simulink model "FaultCheck"  (R2022b)
settings: Solver=FixedStepAuto  StartTime=0.0  StopTime=10  FixedStep=1  RelTol=1e-3
undefined symbols (not defined in the file): C_Flt_IGBTULowerTempConfirmTh_u16, C_Flt_IGBTULowerTempDiagEn_b, C_Flt_IGBTULowerTempErrCode_u16, C_Flt_IGBTULowerTempPowerCoeff, C_Flt_IGBTULowerTempRecoveryTh_u16, C_Flt_IGBTULowerTempRecTh_s32, C_Flt_IGBTULowerTempTrigTh_s32, C_Flt_IGBTUOverTempConfirmTh_u16, C_Flt_IGBTUOverTempDiagEn_b, C_Flt_IGBTUOverTempErrCode_u16, C_Flt_IGBTUOverTempRecoveryTh_u16, C_Flt_IGBTUOverTempRecTh_s32, C_Flt_IGBTUOverTempTrigTh_s32, C_Flt_IGBTVLowerTempConfirmTh_u16, C_Flt_IGBTVLowerTempDiagEn_b, C_Flt_IGBTVLowerTempErrCode_u16, C_Flt_IGBTVLowerTempPowerCoeff, C_Flt_IGBTVLowerTempRecoveryTh_u16, C_Flt_IGBTVLowerTempRecTh_s32, C_Flt_IGBTVLowerTempTrigTh_s32, C_Flt_IGBTVOverTempConfirmTh_u16, C_Flt_IGBTVOverTempDiagEn_b, C_Flt_IGBTVOverTempErrCode_u16, C_Flt_IGBTVOverTempRecoveryTh_u16, C_Flt_IGBTVOverTempRecTh_s32, C_Flt_IGBTVOverTempTrigTh_s32, C_Flt_IGBTWLowerTempConfirmTh_u16, C_Flt_IGBTWLowerTempDiagEn_b, C_Flt_IGBTWLowerTempErrCode_u16, C_Flt_IGBTWLowerTempPowerCoeff, C_Flt_IGBTWLowerTempRecoveryTh_u16, C_Flt_IGBTWLowerTempRecTh_s32, C_Flt_IGBTWLowerTempTrigTh_s32, C_Flt_IGBTWOverTempConfirmTh_u16, C_Flt_IGBTWOverTempDiagEn_b, C_Flt_IGBTWOverTempErrCode_u16, C_Flt_IGBTWOverTempRecoveryTh_u16, C_Flt_IGBTWOverTempRecTh_s32, C_Flt_IGBTWOverTempTrigTh_s32, C_Flt_IuOCConfirmTh_u16, C_Flt_IuOCDiagEn_b, C_Flt_IuOCErrCode_u16, C_Flt_IuOCNegLimit_s32, C_Flt_IuOCPosLimit_s32, C_Flt_IuOCRecoveryTh_u16, C_Flt_IuZeroDriftDiagEn_b, C_Flt_IuZeroDriftErrCode_u16, C_Flt_IvOCConfirmTh_u16, C_Flt_IvOCDiagEn_b, C_Flt_IvOCErrCode_u16, C_Flt_IvOCNegLimit_s32, C_Flt_IvOCPosLimit_s32, C_Flt_IvOCRecoveryTh_u16, C_Flt_IvZeroDriftDiagEn_b, C_Flt_IvZeroDriftErrCode_u16, C_Flt_IwOCConfirmTh_u16, C_Flt_IwOCDiagEn_b, C_Flt_IwOCErrCode_u16, C_Flt_IwOCNegLimit_s32, C_Flt_IwOCPosLimit_s32 ... (+196)
libraries: YS_UserDefined_Library x21, simulink x5
(part 5 of 11)

== system FaultCheck/FaultDiagnose/IGBTTempDiag/IGBTWOverTempDiag/PowerReductionCoeffDeter ==
  IGBTWOverTempFltLevelOut : Inport
  PowerCoeff : Inport  Port=2
  If : If  IfExpression=u1 < 2  ElseIfExpressions=u1 == 2
  If Action Subsystem : Subsystem  TreatAsAtomicUnit=on
  If Action Subsystem1 : Subsystem  TreatAsAtomicUnit=on
  If Action Subsystem2 : Subsystem  TreatAsAtomicUnit=on
  Merge : Merge  Inputs=3
  IGBTWOverTempPowerCoeffOut : Outport
  wires:
  IGBTWOverTempFltLevelOut/1 -> If/1
  If/1 -> If Action Subsystem/Action
  If/2 -> If Action Subsystem1/Action
  If/3 -> If Action Subsystem2/Action
  PowerCoeff/1 -> If Action Subsystem1/1(PowerCoeff)
  If Action Subsystem/1(Coeff) -> Merge/1
  If Action Subsystem1/1(Coeff) -> Merge/2
  If Action Subsystem2/1(Coeff) -> Merge/3
  Merge/1 -> IGBTWOverTempPowerCoeffOut/1  "M_Flt_IGBTWOverTempPowerCoeffOut_s32"

== system FaultCheck/FaultDiagnose/MotorSpdFltDiag/MotorOverSpdOneNegDiag/Diagnose ==
  DiagEnOut : Inport
  MotorSpd : Inport  Port=2
  Parameter : Inport  Port=3
  Disable : Subsystem  TreatAsAtomicUnit=on
  If : If  IfExpression=u1 == 0
  Merge : Merge
  NormalDiag : Subsystem  TreatAsAtomicUnit=on
  MotorOverSpdOneNegFlgOut : Outport
  wires:
  DiagEnOut/1 -> If/1
  If/1 -> Disable/Action
  If/2 -> NormalDiag/Action
  MotorSpd/1 -> NormalDiag/1(MotorSpd)
  Parameter/1 -> NormalDiag/2(Parameter)
  Disable/1(MotorOverSpdOneNegFltDeb) -> Merge/1
  NormalDiag/1(MotorOverSpdOneNegFltDeb) -> Merge/2
  Merge/1 -> MotorOverSpdOneNegFlgOut/1  "M_Flt_MotorOverSpdOneNegFlgOut_b"

== system FaultCheck/FaultDiagnose/MotorSpdFltDiag/MotorOverSpdOneNegDiag/EnableJudgement ==
  SysSelfCheckDownFlg : Inport
  DiagEn : Inport  Port=2
  Constant : Constant  Value=true
  Logical Operator : Logic  AllPortsSameDT=off  OutDataTypeStr=boolean
  Logical Operator1 : Logic  AllPortsSameDT=off  OutDataTypeStr=boolean
  Logical Operator2 : Logic  AllPortsSameDT=off  OutDataTypeStr=boolean
  DiagEnOut : Outport
  wires:
  Logical Operator2/1 -> DiagEnOut/1  "M_Flt_MotorOverSpdOneNegDiagEn_b"
  Logical Operator/1 -> Logical Operator2/1
  SysSelfCheckDownFlg/1 -> Logical Operator/2
  DiagEn/1 -> Logical Operator1/2
  Constant/1 -> Logical Operator/1, Logical Operator1/1
  Logical Operator1/1 -> Logical Operator2/2

== system FaultCheck/FaultDiagnose/MotorSpdFltDiag/MotorOverSpdOneNegDiag/FaultLevelDeter ==
  MotorOverSpdOneNegFlgOut : Inport
  FaultLevel : Inport  Port=2
  If : If  IfExpression=u1 == 0
  LowerOne : Subsystem  TreatAsAtomicUnit=on
  Merge : Merge
  Normal : Subsystem  TreatAsAtomicUnit=on
  MotorOverSpdOneNegFltLevelOut : Outport
  wires:
  MotorOverSpdOneNegFlgOut/1 -> If/1
  If/1 -> Normal/Action
  If/2 -> LowerOne/Action
  Normal/1(MotorOverSpdOneNegFltLevel) -> Merge/1
  LowerOne/1(MotorOverSpdOneNegFltLevel) -> Merge/2
  Merge/1 -> MotorOverSpdOneNegFltLevelOut/1  "M_Flt_MotorOverSpdOneNegFltLevelOut_u8"
  FaultLevel/1 -> LowerOne/1(FaultLevel)

== system FaultCheck/FaultDiagnose/MotorSpdFltDiag/MotorOverSpdOneNegDiag/Parameters ==
  MotorSpd : Inport
  1-D Lookup Table1 : Lookup_n-D  NumberOfTableDimensions=1  BreakpointsForDimension1=[-5:5]  BreakpointsForDimension1DataTypeStr=Inherit: Inherit from 'Breakpoint data'  IndexSearchMethod=Linear search  Table=tanh([-5:5])  TableDataTypeStr=Inherit: Inherit from 'Table data'  ExtrapMethod=Clip  UseLastTableValue=on  InternalRulePriority=Speed  OutDataTypeStr=single  RndMeth=Simplest
  Bus Creator : BusCreator  Inputs=8
  Constant : Constant  Value=C_Flt_MotorOverSpdOneNegTrigTh_s32
  Constant1 : Constant  Value=C_Flt_MotorOverSpdOneNegRecTh_s32
  Constant10 : Constant  Value=C_Flt_MotorOverSpdOneNegRecoveryTh_u16
  Constant11 : Constant  Value=C_Flt_LevelTwo_u8
  Constant7 : Constant  Value=C_Flt_MotorOverSpdOneNegDiagEn_b
  Constant8 : Constant  Value=C_Flt_MotorOverSpdOneNegErrCode_u16
  Constant9 : Constant  Value=C_Flt_MotorOverSpdOneNegConfirmTh_u16
  Param : Outport
  wires:
  Bus Creator/1 -> Param/1
  MotorSpd/1 -> 1-D Lookup Table1/1
  Constant/1 -> Bus Creator/1  "MotorOverSpdOneNegTrigTh"
  Constant7/1 -> Bus Creator/3  "MotorOverSpdOneNegDiagEn"
  Constant8/1 -> Bus Creator/4  "MotorOverSpdOneNegErrCode"
  Constant9/1 -> Bus Creator/5  "MotorOverSpdOneNegConfirmTh"
  Constant10/1 -> Bus Creator/6  "MotorOverSpdOneNegRecoveryTh"
  Constant11/1 -> Bus Creator/7  "MotorOverSpdOneNegFltLevel"
  1-D Lookup Table1/1 -> Bus Creator/8  "MotorOverSpdOneNegPowerCoeff"
  Constant1/1 -> Bus Creator/2  "MotorOverSpdOneNegRecTh"

== system FaultCheck/FaultDiagnose/MotorSpdFltDiag/MotorOverSpdOneNegDiag/PowerReductionCoeffDeter ==
  MotorOverSpdOneNegFltLevelOut : Inport
  PowerCoeff : Inport  Port=2
  If : If  IfExpression=u1 < 2  ElseIfExpressions=u1 == 2
  If Action Subsystem : Subsystem  TreatAsAtomicUnit=on
  If Action Subsystem1 : Subsystem  TreatAsAtomicUnit=on
  If Action Subsystem2 : Subsystem  TreatAsAtomicUnit=on
  Merge : Merge  Inputs=3
  MotorOverSpdOneNegPowerCoeffOut : Outport
  wires:
  MotorOverSpdOneNegFltLevelOut/1 -> If/1
  If/1 -> If Action Subsystem/Action
  If/2 -> If Action Subsystem1/Action
  If/3 -> If Action Subsystem2/Action
  PowerCoeff/1 -> If Action Subsystem1/1(PowerCoeff)
  If Action Subsystem/1(Coeff) -> Merge/1
  If Action Subsystem1/1(Coeff) -> Merge/2
  If Action Subsystem2/1(Coeff) -> Merge/3
  Merge/1 -> MotorOverSpdOneNegPowerCoeffOut/1  "M_Flt_MotorOverSpdOneNegPowerCoeffOut_s32"

== system FaultCheck/FaultDiagnose/MotorSpdFltDiag/MotorOverSpdOnePosDiag/Diagnose ==
  DiagEnOut : Inport
  MotorSpd : Inport  Port=2
  Parameter : Inport  Port=3
  Disable : Subsystem  TreatAsAtomicUnit=on
  If : If  IfExpression=u1 == 0
  Merge : Merge
  NormalDiag : Subsystem  TreatAsAtomicUnit=on
  MotorOverSpdOnePosFlgOut : Outport
  wires:
  DiagEnOut/1 -> If/1
  If/1 -> Disable/Action
  If/2 -> NormalDiag/Action
  MotorSpd/1 -> NormalDiag/1(MotorSpd)
  Parameter/1 -> NormalDiag/2(Parameter)
  Disable/1(MotorOverSpdOnePosFltDeb) -> Merge/1
  NormalDiag/1(MotorOverSpdOnePosFltDeb) -> Merge/2
  Merge/1 -> MotorOverSpdOnePosFlgOut/1  "M_Flt_MotorOverSpdOnePosFlgOut_b"

== system FaultCheck/FaultDiagnose/MotorSpdFltDiag/MotorOverSpdOnePosDiag/EnableJudgement ==
  SysSelfCheckDownFlg : Inport
  DiagEn : Inport  Port=2
  Constant : Constant  Value=true
  Logical Operator : Logic  AllPortsSameDT=off  OutDataTypeStr=boolean
  Logical Operator1 : Logic  AllPortsSameDT=off  OutDataTypeStr=boolean
  Logical Operator2 : Logic  AllPortsSameDT=off  OutDataTypeStr=boolean
  DiagEnOut : Outport
  wires:
  Logical Operator2/1 -> DiagEnOut/1  "M_Flt_MotorOverSpdOnePosDiagEn_b"
  Logical Operator/1 -> Logical Operator2/1
  SysSelfCheckDownFlg/1 -> Logical Operator/2
  DiagEn/1 -> Logical Operator1/2
  Constant/1 -> Logical Operator/1, Logical Operator1/1
  Logical Operator1/1 -> Logical Operator2/2

== system FaultCheck/FaultDiagnose/MotorSpdFltDiag/MotorOverSpdOnePosDiag/FaultLevelDeter ==
  MotorOverSpdOnePosFlgOut : Inport
  FaultLevel : Inport  Port=2
  If : If  IfExpression=u1 == 0
  LowerOne : Subsystem  TreatAsAtomicUnit=on
  Merge : Merge
  Normal : Subsystem  TreatAsAtomicUnit=on
  MotorOverSpdOnePosFltLevelOut : Outport
  wires:
  MotorOverSpdOnePosFlgOut/1 -> If/1
  If/1 -> Normal/Action
  If/2 -> LowerOne/Action
  Normal/1(MotorOverSpdOnePosFltLevel) -> Merge/1
  LowerOne/1(MotorOverSpdOnePosFltLevel) -> Merge/2
  Merge/1 -> MotorOverSpdOnePosFltLevelOut/1  "M_Flt_MotorOverSpdOnePosFltLevelOut_u8"
  FaultLevel/1 -> LowerOne/1(FaultLevel)

== system FaultCheck/FaultDiagnose/MotorSpdFltDiag/MotorOverSpdOnePosDiag/Parameters ==
  MotorSpd : Inport
  1-D Lookup Table1 : Lookup_n-D  NumberOfTableDimensions=1  BreakpointsForDimension1=[-5:5]  BreakpointsForDimension1DataTypeStr=Inherit: Inherit from 'Breakpoint data'  IndexSearchMethod=Linear search  Table=tanh([-5:5])  TableDataTypeStr=Inherit: Inherit from 'Table data'  ExtrapMethod=Clip  UseLastTableValue=on  InternalRulePriority=Speed  OutDataTypeStr=single  RndMeth=Simplest
  Bus Creator : BusCreator  Inputs=8
  Constant : Constant  Value=C_Flt_MotorOverSpdOnePosTrigTh_s32
  Constant1 : Constant  Value=C_Flt_MotorOverSpdOnePosRecTh_s32
  Constant10 : Constant  Value=C_Flt_MotorOverSpdOnePosRecoveryTh_u16
  Constant11 : Constant  Value=C_Flt_LevelTwo_u8
  Constant7 : Constant  Value=C_Flt_MotorOverSpdOnePosDiagEn_b
  Constant8 : Constant  Value=C_Flt_MotorOverSpdOnePosErrCode_u16
  Constant9 : Constant  Value=C_Flt_MotorOverSpdOnePosConfirmTh_u16
  Param : Outport
  wires:
  Bus Creator/1 -> Param/1
  MotorSpd/1 -> 1-D Lookup Table1/1
  Constant/1 -> Bus Creator/1  "MotorOverSpdOnePosTrigTh"
  Constant7/1 -> Bus Creator/3  "MotorOverSpdOnePosDiagEn"
  Constant8/1 -> Bus Creator/4  "MotorOverSpdOnePosErrCode"
  Constant9/1 -> Bus Creator/5  "MotorOverSpdOnePosConfirmTh"
  Constant10/1 -> Bus Creator/6  "MotorOverSpdOnePosRecoveryTh"
  Constant11/1 -> Bus Creator/7  "MotorOverSpdOnePosFltLevel"
  1-D Lookup Table1/1 -> Bus Creator/8  "MotorOverSpdOnePosPowerCoeff"
  Constant1/1 -> Bus Creator/2  "MotorOverSpdOnePosRecTh"

== system FaultCheck/FaultDiagnose/MotorSpdFltDiag/MotorOverSpdOnePosDiag/PowerReductionCoeffDeter ==
  MotorOverSpdOnePosFltLevelOut : Inport
  PowerCoeff : Inport  Port=2
  If : If  IfExpression=u1 < 2  ElseIfExpressions=u1 == 2
  If Action Subsystem : Subsystem  TreatAsAtomicUnit=on
  If Action Subsystem1 : Subsystem  TreatAsAtomicUnit=on
  If Action Subsystem2 : Subsystem  TreatAsAtomicUnit=on
  Merge : Merge  Inputs=3
  MotorOverSpdOnePosPowerCoeffOut : Outport
  wires:
  MotorOverSpdOnePosFltLevelOut/1 -> If/1
  If/1 -> If Action Subsystem/Action
  If/2 -> If Action Subsystem1/Action
  If/3 -> If Action Subsystem2/Action
  PowerCoeff/1 -> If Action Subsystem1/1(PowerCoeff)
  If Action Subsystem/1(Coeff) -> Merge/1
  If Action Subsystem1/1(Coeff) -> Merge/2
  If Action Subsystem2/1(Coeff) -> Merge/3
  Merge/1 -> MotorOverSpdOnePosPowerCoeffOut/1  "M_Flt_MotorOverSpdOnePosPowerCoeffOut_s32"

== system FaultCheck/FaultDiagnose/MotorSpdFltDiag/MotorOverSpdTwoNegDiag/Diagnose ==
  DiagEnOut : Inport
  MotorSpd : Inport  Port=2
  Parameter : Inport  Port=3
  Disable : Subsystem  TreatAsAtomicUnit=on
  If : If  IfExpression=u1 == 0
  Merge : Merge
  NormalDiag : Subsystem  TreatAsAtomicUnit=on
  MotorOverSpdTwoNegFlgOut : Outport
  wires:
  Merge/1 -> MotorOverSpdTwoNegFlgOut/1  "M_Flt_MotorOverSpdTwoNegFlgOut_b"
  NormalDiag/1(MotorOverSpdTwoNegFltDeb) -> Merge/2
  Disable/1(MotorOverSpdTwoNegFltDeb) -> Merge/1
  Parameter/1 -> NormalDiag/2(Parameter)
  MotorSpd/1 -> NormalDiag/1(PCBTemp)
  If/2 -> NormalDiag/Action
  If/1 -> Disable/Action
  DiagEnOut/1 -> If/1

== system FaultCheck/FaultDiagnose/MotorSpdFltDiag/MotorOverSpdTwoNegDiag/EnableJudgement ==
  SysSelfCheckDownFlg : Inport
  DiagEn : Inport  Port=2
  Constant : Constant  Value=true
  Logical Operator : Logic  AllPortsSameDT=off  OutDataTypeStr=boolean
  Logical Operator1 : Logic  AllPortsSameDT=off  OutDataTypeStr=boolean
  Logical Operator2 : Logic  AllPortsSameDT=off  OutDataTypeStr=boolean
  DiagEnOut : Outport
  wires:
  Logical Operator1/1 -> Logical Operator2/2
  Constant/1 -> Logical Operator1/1, Logical Operator/1
  DiagEn/1 -> Logical Operator1/2
  SysSelfCheckDownFlg/1 -> Logical Operator/2
  Logical Operator/1 -> Logical Operator2/1
  Logical Operator2/1 -> DiagEnOut/1  "M_Flt_MotorOverSpdTwoNegDiagEn_b"

== system FaultCheck/FaultDiagnose/MotorSpdFltDiag/MotorOverSpdTwoNegDiag/FaultLevelDeter ==
  MotorOverSpdTwoNegFlgOut : Inport
  FaultLevel : Inport  Port=2
  If : If  IfExpression=u1 == 0
  LowerOne : Subsystem  TreatAsAtomicUnit=on
  Merge : Merge
  Normal : Subsystem  TreatAsAtomicUnit=on
  MotorOverSpdTwoNegFltLevelOut : Outport
  wires:
  FaultLevel/1 -> LowerOne/1(FaultLevel)
  Merge/1 -> MotorOverSpdTwoNegFltLevelOut/1  "M_Flt_MotorOverSpdTwoNegFltLevelOut_u8"
  LowerOne/1(MotorOverSpdTwoNegFltLevel) -> Merge/2
  Normal/1(MotorOverSpdTwoNegFltLevel) -> Merge/1
  If/2 -> LowerOne/Action
  If/1 -> Normal/Action
  MotorOverSpdTwoNegFlgOut/1 -> If/1

== system FaultCheck/FaultDiagnose/MotorSpdFltDiag/MotorOverSpdTwoNegDiag/Parameters ==
  Bus Creator : BusCreator  Inputs=8
  Constant : Constant  Value=C_Flt_MotorOverSpdTwoNegTrigTh_s32
  Constant1 : Constant  Value=C_Flt_MotorOverSpdTwoNegRecTh_s32
  Constant10 : Constant  Value=C_Flt_MotorOverSpdTwoNegRecoveryTh_u16
  Constant11 : Constant  Value=C_Flt_LevelThree_u8
  Constant2 : Constant  Value=C_Flt_PowerCoeffZero_s32
  Constant7 : Constant  Value=C_Flt_MotorOverSpdTwoNegDiagEn_b
  Constant8 : Constant  Value=C_Flt_MotorOverSpdTwoNegErrCode_u16
  Constant9 : Constant  Value=C_Flt_MotorOverSpdTwoNegConfirmTh_u16
  Param : Outport
  wires:
  Constant1/1 -> Bus Creator/2  "MotorOverSpdTwoNegRecTh"
  Constant2/1 -> Bus Creator/8  "MotorOverSpdTwoNegPowerCoeff"
  Constant11/1 -> Bus Creator/7  "MotorOverSpdTwoNegFltLevel"
  Constant10/1 -> Bus Creator/6  "MotorOverSpdTwoNegRecoveryTh"
  Constant9/1 -> Bus Creator/5  "MotorOverSpdTwoNegConfirmTh"
  Constant8/1 -> Bus Creator/4  "MotorOverSpdTwoNegErrCode"
  Constant7/1 -> Bus Creator/3  "MotorOverSpdTwoNegDiagEn"
  Constant/1 -> Bus Creator/1  "MotorOverSpdTwoNegTrigTh"
  Bus Creator/1 -> Param/1

== system FaultCheck/FaultDiagnose/MotorSpdFltDiag/MotorOverSpdTwoNegDiag/PowerReductionCoeffDeter ==
  MotorOverSpdTwoNegFltLevelOut : Inport
  PowerCoeff : Inport  Port=2
  If : If  IfExpression=u1 < 2  ElseIfExpressions=u1 == 2
  If Action Subsystem : Subsystem  TreatAsAtomicUnit=on
  If Action Subsystem1 : Subsystem  TreatAsAtomicUnit=on
  If Action Subsystem2 : Subsystem  TreatAsAtomicUnit=on
  Merge : Merge  Inputs=3
  MotorOverSpdTwoNegPowerCoeffOut : Outport
  wires:
  Merge/1 -> MotorOverSpdTwoNegPowerCoeffOut/1  "M_Flt_MotorOverSpdTwoNegPowerCoeffOut_s32"
  If Action Subsystem2/1(Coeff) -> Merge/3
  If Action Subsystem1/1(Coeff) -> Merge/2
  If Action Subsystem/1(Coeff) -> Merge/1
  PowerCoeff/1 -> If Action Subsystem1/1(PowerCoeff)
  If/3 -> If Action Subsystem2/Action
  If/2 -> If Action Subsystem1/Action
  If/1 -> If Action Subsystem/Action
  MotorOverSpdTwoNegFltLevelOut/1 -> If/1

== system FaultCheck/FaultDiagnose/MotorSpdFltDiag/MotorOverSpdTwoPosDiag/Diagnose ==
  DiagEnOut : Inport
  MotorSpd : Inport  Port=2
  Parameter : Inport  Port=3
  Disable : Subsystem  TreatAsAtomicUnit=on
  If : If  IfExpression=u1 == 0
  Merge : Merge
  NormalDiag : Subsystem  TreatAsAtomicUnit=on
  MotorOverSpdTwoPosFlgOut : Outport
  wires:
  Merge/1 -> MotorOverSpdTwoPosFlgOut/1  "M_Flt_MotorOverSpdTwoPosFlgOut_b"
  NormalDiag/1(MotorOverSpdTwoPosFltDeb) -> Merge/2
  Disable/1(MotorOverSpdTwoPosFltDeb) -> Merge/1
  Parameter/1 -> NormalDiag/2(Parameter)
  MotorSpd/1 -> NormalDiag/1(MotorSpd)
  If/2 -> NormalDiag/Action
  If/1 -> Disable/Action
  DiagEnOut/1 -> If/1

== system FaultCheck/FaultDiagnose/MotorSpdFltDiag/MotorOverSpdTwoPosDiag/EnableJudgement ==
  SysSelfCheckDownFlg : Inport
  DiagEn : Inport  Port=2
  Constant : Constant  Value=true
  Logical Operator : Logic  AllPortsSameDT=off  OutDataTypeStr=boolean
  Logical Operator1 : Logic  AllPortsSameDT=off  OutDataTypeStr=boolean
  Logical Operator2 : Logic  AllPortsSameDT=off  OutDataTypeStr=boolean
  DiagEnOut : Outport
  wires:
  Logical Operator1/1 -> Logical Operator2/2
  Constant/1 -> Logical Operator1/1, Logical Operator/1
  DiagEn/1 -> Logical Operator1/2
  SysSelfCheckDownFlg/1 -> Logical Operator/2
  Logical Operator/1 -> Logical Operator2/1
  Logical Operator2/1 -> DiagEnOut/1  "M_Flt_MotorOverSpdTwoPosDiagEn_b"

== system FaultCheck/FaultDiagnose/MotorSpdFltDiag/MotorOverSpdTwoPosDiag/FaultLevelDeter ==
  MotorOverSpdTwoPosFlgOut : Inport
  FaultLevel : Inport  Port=2
  If : If  IfExpression=u1 == 0
  LowerOne : Subsystem  TreatAsAtomicUnit=on
  Merge : Merge
  Normal : Subsystem  TreatAsAtomicUnit=on
  MotorOverSpdTwoPosFltLevelOut : Outport
  wires:
  FaultLevel/1 -> LowerOne/1(FaultLevel)
  Merge/1 -> MotorOverSpdTwoPosFltLevelOut/1  "M_Flt_MotorOverSpdTwoPosFltLevelOut_u8"
  LowerOne/1(MotorOverSpdTwoPosFltLevel) -> Merge/2
  Normal/1(MotorOverSpdTwoPosFltLevel) -> Merge/1
  If/2 -> LowerOne/Action
  If/1 -> Normal/Action
  MotorOverSpdTwoPosFlgOut/1 -> If/1

== system FaultCheck/FaultDiagnose/MotorSpdFltDiag/MotorOverSpdTwoPosDiag/Parameters ==
  Bus Creator : BusCreator  Inputs=8
  Constant : Constant  Value=C_Flt_MotorOverSpdTwoPosTrigTh_s32
  Constant1 : Constant  Value=C_Flt_MotorOverSpdTwoPosRecTh_s32
  Constant10 : Constant  Value=C_Flt_MotorOverSpdTwoPosRecoveryTh_u16
  Constant11 : Constant  Value=C_Flt_LevelThree_u8
  Constant2 : Constant  Value=C_Flt_PowerCoeffZero_s32
  Constant7 : Constant  Value=C_Flt_MotorOverSpdTwoPosDiagEn_b
  Constant8 : Constant  Value=C_Flt_MotorOverSpdTwoPosErrCode_u16
  Constant9 : Constant  Value=C_Flt_MotorOverSpdTwoPosConfirmTh_u16
  Param : Outport
  wires:
  Constant1/1 -> Bus Creator/2  "MotorOverSpdTwoPosRecTh"
  Constant2/1 -> Bus Creator/8  "MotorOverSpdTwoPosPowerCoeff"
  Constant11/1 -> Bus Creator/7  "MotorOverSpdTwoPosFltLevel"
  Constant10/1 -> Bus Creator/6  "MotorOverSpdTwoPosRecoveryTh"
  Constant9/1 -> Bus Creator/5  "MotorOverSpdTwoPosConfirmTh"
  Constant8/1 -> Bus Creator/4  "MotorOverSpdTwoPosErrCode"
  Constant7/1 -> Bus Creator/3  "MotorOverSpdTwoPosDiagEn"
  Constant/1 -> Bus Creator/1  "MotorOverSpdTwoPosTrigTh"
  Bus Creator/1 -> Param/1

== system FaultCheck/FaultDiagnose/MotorSpdFltDiag/MotorOverSpdTwoPosDiag/PowerReductionCoeffDeter ==
  MotorOverSpdTwoPosFltLevelOut : Inport
  PowerCoeff : Inport  Port=2
  If : If  IfExpression=u1 < 2  ElseIfExpressions=u1 == 2
  If Action Subsystem : Subsystem  TreatAsAtomicUnit=on
  If Action Subsystem1 : Subsystem  TreatAsAtomicUnit=on
  If Action Subsystem2 : Subsystem  TreatAsAtomicUnit=on
  Merge : Merge  Inputs=3
  MotorOverSpdTwoPosPowerCoeffOut : Outport
  wires:
  Merge/1 -> MotorOverSpdTwoPosPowerCoeffOut/1  "M_Flt_MotorOverSpdTwoPosPowerCoeffOut_s32"
  If Action Subsystem2/1(Coeff) -> Merge/3
  If Action Subsystem1/1(Coeff) -> Merge/2
  If Action Subsystem/1(Coeff) -> Merge/1
  PowerCoeff/1 -> If Action Subsystem1/1(PowerCoeff)
  If/3 -> If Action Subsystem2/Action
  If/2 -> If Action Subsystem1/Action
  If/1 -> If Action Subsystem/Action
  MotorOverSpdTwoPosFltLevelOut/1 -> If/1

== system FaultCheck/FaultDiagnose/MotorTempDiag/MotorLowerTempDiag/Diagnose ==
  DiagEnOut : Inport
  MotorTemp : Inport  Port=2
  Parameter : Inport  Port=3
  Disable : Subsystem  TreatAsAtomicUnit=on
  If : If  IfExpression=u1 == 0
  Merge : Merge
  NormalDiag : Subsystem  TreatAsAtomicUnit=on
  MotorLowerTempFlgOut : Outport
  wires:
  Merge/1 -> MotorLowerTempFlgOut/1  "M_Flt_MotorLowerTempFlgOut_b"
  NormalDiag/1(MotorLowerTempFltDeb) -> Merge/2
  Disable/1(MotorLowerTempFltDeb) -> Merge/1
  Parameter/1 -> NormalDiag/2(Parameter)
  MotorTemp/1 -> NormalDiag/1(MotorTemp)
  If/2 -> NormalDiag/Action
  If/1 -> Disable/Action
  DiagEnOut/1 -> If/1

== system FaultCheck/FaultDiagnose/MotorTempDiag/MotorLowerTempDiag/EnableJudgement ==
  SysSelfCheckDownFlg : Inport
  DiagEn : Inport  Port=2
  Constant : Constant  Value=true
  Logical Operator : Logic  AllPortsSameDT=off  OutDataTypeStr=boolean
  Logical Operator1 : Logic  AllPortsSameDT=off  OutDataTypeStr=boolean
  Logical Operator2 : Logic  AllPortsSameDT=off  OutDataTypeStr=boolean
  DiagEnOut : Outport
  wires:
  Logical Operator1/1 -> Logical Operator2/2
  Constant/1 -> Logical Operator1/1, Logical Operator/1
  DiagEn/1 -> Logical Operator1/2
  SysSelfCheckDownFlg/1 -> Logical Operator/2
  Logical Operator/1 -> Logical Operator2/1
  Logical Operator2/1 -> DiagEnOut/1  "M_Flt_MotorLowerTempDiagEn_b"

== system FaultCheck/FaultDiagnose/MotorTempDiag/MotorLowerTempDiag/FaultLevelDeter ==
  MotorLowerTempFlgOut : Inport
  FaultLevel : Inport  Port=2
  If : If  IfExpression=u1 == 0
  LowerOne : Subsystem  TreatAsAtomicUnit=on
  Merge : Merge
  Normal : Subsystem  TreatAsAtomicUnit=on
  MotorLowerTempFltLevelOut : Outport
  wires:
  FaultLevel/1 -> LowerOne/1(FaultLevel)
  Merge/1 -> MotorLowerTempFltLevelOut/1  "M_Flt_MotorLowerTempFltLevelOut_u8"
  LowerOne/1(MotorLowerTempFltLevel) -> Merge/2
  Normal/1(MotorLowerTempFltLevel) -> Merge/1
  If/2 -> LowerOne/Action
  If/1 -> Normal/Action
  MotorLowerTempFlgOut/1 -> If/1

== system FaultCheck/FaultDiagnose/MotorTempDiag/MotorLowerTempDiag/Parameters ==
  Bus Creator : BusCreator  Inputs=8
  Constant : Constant  Value=C_Flt_MotorLowerTempTrigTh_s32
  Constant1 : Constant  Value=C_Flt_MotorLowerTempRecTh_s32
  Constant10 : Constant  Value=C_Flt_MotorLowerTempRecoveryTh_u16
  Constant11 : Constant  Value=C_Flt_LevelTwo_u8
  Constant2 : Constant  Value=C_Flt_MotorLowerTempPowerCoeff
  Constant7 : Constant  Value=C_Flt_MotorLowerTempDiagEn_b
  Constant8 : Constant  Value=C_Flt_MotorLowerTempErrCode_u16
  Constant9 : Constant  Value=C_Flt_MotorLowerTempConfirmTh_u16
  Param : Outport
  wires:
  Constant1/1 -> Bus Creator/2  "MotorLowerTempRecTh"
  Constant2/1 -> Bus Creator/8  "MotorLowerTempPowerCoeff"
  Constant11/1 -> Bus Creator/7  "MotorLowerTempFltLevel"
  Constant10/1 -> Bus Creator/6  "MotorLowerTempRecoveryTh"
  Constant9/1 -> Bus Creator/5  "MotorLowerTempConfirmTh"
  Constant8/1 -> Bus Creator/4  "MotorLowerTempErrCode"
  Constant7/1 -> Bus Creator/3  "MotorLowerTempDiagEn"
  Constant/1 -> Bus Creator/1  "MotorLowerTempTrigTh"
  Bus Creator/1 -> Param/1

== system FaultCheck/FaultDiagnose/MotorTempDiag/MotorLowerTempDiag/PowerReductionCoeffDeter ==
  MotorLowerTempFltLevelOut : Inport
  PowerCoeff : Inport  Port=2
  If : If  IfExpression=u1 < 2  ElseIfExpressions=u1 == 2
  If Action Subsystem : Subsystem  TreatAsAtomicUnit=on
  If Action Subsystem1 : Subsystem  TreatAsAtomicUnit=on
  If Action Subsystem2 : Subsystem  TreatAsAtomicUnit=on
  Merge : Merge  Inputs=3
  MotorLowerTempPowerCoeffOut : Outport
  wires:
  Merge/1 -> MotorLowerTempPowerCoeffOut/1  "M_Flt_MotorLowerTempPowerCoeffOut_s32"
  If Action Subsystem2/1(Coeff) -> Merge/3
  If Action Subsystem1/1(Coeff) -> Merge/2
  If Action Subsystem/1(Coeff) -> Merge/1
  PowerCoeff/1 -> If Action Subsystem1/1(PowerCoeff)
  If/3 -> If Action Subsystem2/Action
  If/2 -> If Action Subsystem1/Action
  If/1 -> If Action Subsystem/Action
  MotorLowerTempFltLevelOut/1 -> If/1

== system FaultCheck/FaultDiagnose/MotorTempDiag/MotorOverTempDiag/Diagnose ==
  DiagEnOut : Inport
  MotorTemp : Inport  Port=2
  Parameter : Inport  Port=3
  Disable : Subsystem  TreatAsAtomicUnit=on
  If : If  IfExpression=u1 == 0
  Merge : Merge
  NormalDiag : Subsystem  TreatAsAtomicUnit=on
  MotorOverTempFlgOut : Outport
  wires:
  DiagEnOut/1 -> If/1
  If/1 -> Disable/Action
  If/2 -> NormalDiag/Action
  MotorTemp/1 -> NormalDiag/1(MotorTemp)
  Parameter/1 -> NormalDiag/2(Parameter)
  Disable/1(MotorOverTempFltDeb) -> Merge/1
  NormalDiag/1(MotorOverTempFltDeb) -> Merge/2
  Merge/1 -> MotorOverTempFlgOut/1  "M_Flt_MotorOverTempFlgOut_b"

== system FaultCheck/FaultDiagnose/MotorTempDiag/MotorOverTempDiag/EnableJudgement ==
  SysSelfCheckDownFlg : Inport
  DiagEn : Inport  Port=2
  Constant : Constant  Value=true
  Logical Operator : Logic  AllPortsSameDT=off  OutDataTypeStr=boolean
  Logical Operator1 : Logic  AllPortsSameDT=off  OutDataTypeStr=boolean
  Logical Operator2 : Logic  AllPortsSameDT=off  OutDataTypeStr=boolean
  DiagEnOut : Outport
  wires:
  Logical Operator2/1 -> DiagEnOut/1  "M_Flt_MotorOverTempDiagEn_b"
  Logical Operator/1 -> Logical Operator2/1
  SysSelfCheckDownFlg/1 -> Logical Operator/2
  DiagEn/1 -> Logical Operator1/2
  Constant/1 -> Logical Operator/1, Logical Operator1/1
  Logical Operator1/1 -> Logical Operator2/2

== system FaultCheck/FaultDiagnose/MotorTempDiag/MotorOverTempDiag/FaultLevelDeter ==
  MotorOverTempFlgOut : Inport
  FaultLevel : Inport  Port=2
  If : If  IfExpression=u1 == 0
  LowerOne : Subsystem  TreatAsAtomicUnit=on
  Merge : Merge
  Normal : Subsystem  TreatAsAtomicUnit=on
  MotorOverTempFltLevelOut : Outport
  wires:
  MotorOverTempFlgOut/1 -> If/1
  If/1 -> Normal/Action
  If/2 -> LowerOne/Action
  Normal/1(MotorOverTempFltLevel) -> Merge/1
  LowerOne/1(MotorOverTempFltLevel) -> Merge/2
  Merge/1 -> MotorOverTempFltLevelOut/1  "M_Flt_MotorOverTempFltLevelOut_u8"
  FaultLevel/1 -> LowerOne/1(FaultLevel)

== system FaultCheck/FaultDiagnose/MotorTempDiag/MotorOverTempDiag/Parameters ==
  MotorTemp : Inport
  1-D Lookup Table1 : Lookup_n-D  NumberOfTableDimensions=1  BreakpointsForDimension1=[-5:5]  BreakpointsForDimension1DataTypeStr=Inherit: Inherit from 'Breakpoint data'  IndexSearchMethod=Linear search  Table=tanh([-5:5])  TableDataTypeStr=Inherit: Inherit from 'Table data'  ExtrapMethod=Clip  UseLastTableValue=on  InternalRulePriority=Speed  OutDataTypeStr=single  RndMeth=Simplest
  Bus Creator : BusCreator  Inputs=8
  Constant : Constant  Value=C_Flt_MotorOverTempTrigTh_s32
  Constant1 : Constant  Value=C_Flt_MotorOverTempRecTh_s32
  Constant10 : Constant  Value=C_Flt_MotorOverTempRecoveryTh_u16
  Constant11 : Constant  Value=C_Flt_LevelTwo_u8
  Constant7 : Constant  Value=C_Flt_MotorOverTempDiagEn_b
  Constant8 : Constant  Value=C_Flt_MotorOverTempErrCode_u16
  Constant9 : Constant  Value=C_Flt_MotorOverTempConfirmTh_u16
  Param : Outport
  wires:
  Bus Creator/1 -> Param/1
  MotorTemp/1 -> 1-D Lookup Table1/1
  Constant/1 -> Bus Creator/1  "MotorOverTempTrigTh"
  Constant7/1 -> Bus Creator/3  "MotorOverTempDiagEn"
  Constant8/1 -> Bus Creator/4  "MotorOverTempErrCode"
  Constant9/1 -> Bus Creator/5  "MotorOverTempConfirmTh"
  Constant10/1 -> Bus Creator/6  "MotorOverTempRecoveryTh"
  Constant11/1 -> Bus Creator/7  "MotorOverTempFltLevel"
  1-D Lookup Table1/1 -> Bus Creator/8  "MotorOverTempPowerCoeff"
  Constant1/1 -> Bus Creator/2  "MotorOverTempRecTh"

== system FaultCheck/FaultDiagnose/MotorTempDiag/MotorOverTempDiag/PowerReductionCoeffDeter ==
  MotorOverTempFltLevelOut : Inport
  PowerCoeff : Inport  Port=2
  If : If  IfExpression=u1 < 2  ElseIfExpressions=u1 == 2
  If Action Subsystem : Subsystem  TreatAsAtomicUnit=on
  If Action Subsystem1 : Subsystem  TreatAsAtomicUnit=on
  If Action Subsystem2 : Subsystem  TreatAsAtomicUnit=on
  Merge : Merge  Inputs=3
  MotorOverTempPowerCoeffOut : Outport
  wires:
  MotorOverTempFltLevelOut/1 -> If/1
  If/1 -> If Action Subsystem/Action
  If/2 -> If Action Subsystem1/Action
  If/3 -> If Action Subsystem2/Action
  PowerCoeff/1 -> If Action Subsystem1/1(PowerCoeff)
  If Action Subsystem/1(Coeff) -> Merge/1
  If Action Subsystem1/1(Coeff) -> Merge/2
  If Action Subsystem2/1(Coeff) -> Merge/3
  Merge/1 -> MotorOverTempPowerCoeffOut/1  "M_Flt_MotorOverTempPowerCoeffOut_s32"

== system FaultCheck/FaultDiagnose/PCBTempDiag/PCBLowerTempDiag/Diagnose ==
  DiagEnOut : Inport
  PCBTemp : Inport  Port=2
  Parameter : Inport  Port=3
  Disable : Subsystem  TreatAsAtomicUnit=on
  If : If  IfExpression=u1 == 0
  Merge : Merge
  NormalDiag : Subsystem  TreatAsAtomicUnit=on
  PCBLowerTempFlgOut : Outport
  wires:
  Merge/1 -> PCBLowerTempFlgOut/1  "M_Flt_PCBLowerTempFlgOut_b"
  NormalDiag/1(PCBLowerTempFltDeb) -> Merge/2
  Disable/1(PCBLowerTempFltDeb) -> Merge/1
  Parameter/1 -> NormalDiag/2(Parameter)
  PCBTemp/1 -> NormalDiag/1(PCBTemp)
  If/2 -> NormalDiag/Action
  If/1 -> Disable/Action
  DiagEnOut/1 -> If/1

== system FaultCheck/FaultDiagnose/PCBTempDiag/PCBLowerTempDiag/EnableJudgement ==
  SysSelfCheckDownFlg : Inport
  DiagEn : Inport  Port=2
  Constant : Constant  Value=true
  Logical Operator : Logic  AllPortsSameDT=off  OutDataTypeStr=boolean
  Logical Operator1 : Logic  AllPortsSameDT=off  OutDataTypeStr=boolean
  Logical Operator2 : Logic  AllPortsSameDT=off  OutDataTypeStr=boolean
  DiagEnOut : Outport
  wires:
  Logical Operator1/1 -> Logical Operator2/2
  Constant/1 -> Logical Operator1/1, Logical Operator/1
  DiagEn/1 -> Logical Operator1/2
  SysSelfCheckDownFlg/1 -> Logical Operator/2
  Logical Operator/1 -> Logical Operator2/1
  Logical Operator2/1 -> DiagEnOut/1  "M_Flt_PCBLowerTempDiagEn_b"

== system FaultCheck/FaultDiagnose/PCBTempDiag/PCBLowerTempDiag/FaultLevelDeter ==
  PCBLowerTempFlgOut : Inport
  FaultLevel : Inport  Port=2
  If : If  IfExpression=u1 == 0
  LowerOne : Subsystem  TreatAsAtomicUnit=on
  Merge : Merge
  Normal : Subsystem  TreatAsAtomicUnit=on
  PCBLowerTempFltLevelOut : Outport
  wires:
  FaultLevel/1 -> LowerOne/1(FaultLevel)
  Merge/1 -> PCBLowerTempFltLevelOut/1  "M_Flt_PCBLowerTempFltLevelOut_u8"
  LowerOne/1(PCBLowerTempFltLevel) -> Merge/2
  Normal/1(PCBLowerTempFltLevel) -> Merge/1
  If/2 -> LowerOne/Action
  If/1 -> Normal/Action
  PCBLowerTempFlgOut/1 -> If/1

== system FaultCheck/FaultDiagnose/PCBTempDiag/PCBLowerTempDiag/Parameters ==
  Bus Creator : BusCreator  Inputs=8
  Constant : Constant  Value=C_Flt_PCBLowerTempTrigTh_s32
  Constant1 : Constant  Value=C_Flt_PCBLowerTempRecTh_s32
  Constant10 : Constant  Value=C_Flt_PCBLowerTempRecoveryTh_u16
  Constant11 : Constant  Value=C_Flt_LevelTwo_u8
  Constant2 : Constant  Value=C_Flt_PCBLowerTempPowerCoeff
  Constant7 : Constant  Value=C_Flt_PCBLowerTempDiagEn_b
  Constant8 : Constant  Value=C_Flt_PCBLowerTempErrCode_u16
  Constant9 : Constant  Value=C_Flt_PCBLowerTempConfirmTh_u16
  Param : Outport
  wires:
  Constant1/1 -> Bus Creator/2  "PCBLowerTempRecTh"
  Constant2/1 -> Bus Creator/8  "PCBLowerTempPowerCoeff"
  Constant11/1 -> Bus Creator/7  "PCBLowerTempFltLevel"
  Constant10/1 -> Bus Creator/6  "PCBLowerTempRecoveryTh"
  Constant9/1 -> Bus Creator/5  "PCBLowerTempConfirmTh"
  Constant8/1 -> Bus Creator/4  "PCBLowerTempErrCode"
  Constant7/1 -> Bus Creator/3  "PCBLowerTempDiagEn"
  Constant/1 -> Bus Creator/1  "PCBLowerTempTrigTh"
  Bus Creator/1 -> Param/1

== system FaultCheck/FaultDiagnose/PCBTempDiag/PCBLowerTempDiag/PowerReductionCoeffDeter ==
  PCBLowerTempFltLevelOut : Inport
  PowerCoeff : Inport  Port=2
  If : If  IfExpression=u1 < 2  ElseIfExpressions=u1 == 2
  If Action Subsystem : Subsystem  TreatAsAtomicUnit=on
  If Action Subsystem1 : Subsystem  TreatAsAtomicUnit=on
  If Action Subsystem2 : Subsystem  TreatAsAtomicUnit=on
  Merge : Merge  Inputs=3
  PCBLowerTempPowerCoeffOut : Outport
  wires:
  Merge/1 -> PCBLowerTempPowerCoeffOut/1  "M_Flt_PCBLowerTempPowerCoeffOut_s32"
  If Action Subsystem2/1(Coeff) -> Merge/3
  If Action Subsystem1/1(Coeff) -> Merge/2
  If Action Subsystem/1(Coeff) -> Merge/1
  PowerCoeff/1 -> If Action Subsystem1/1(PowerCoeff)
  If/3 -> If Action Subsystem2/Action
  If/2 -> If Action Subsystem1/Action
  If/1 -> If Action Subsystem/Action
  PCBLowerTempFltLevelOut/1 -> If/1

== system FaultCheck/FaultDiagnose/PCBTempDiag/PCBOverTempDiag/Diagnose ==
  DiagEnOut : Inport
  PCBTemp : Inport  Port=2
  Parameter : Inport  Port=3
  Disable : Subsystem  TreatAsAtomicUnit=on
  If : If  IfExpression=u1 == 0
  Merge : Merge
  NormalDiag : Subsystem  TreatAsAtomicUnit=on
  PCBOverTempFlgOut : Outport
  wires:
  DiagEnOut/1 -> If/1
  If/1 -> Disable/Action
  If/2 -> NormalDiag/Action
  PCBTemp/1 -> NormalDiag/1(PCBTemp)
  Parameter/1 -> NormalDiag/2(Parameter)
  Disable/1(PCBOverTempFltDeb) -> Merge/1
  NormalDiag/1(PCBOverTempFltDeb) -> Merge/2
  Merge/1 -> PCBOverTempFlgOut/1  "M_Flt_PCBOverTempFlgOut_b"

== system FaultCheck/FaultDiagnose/PCBTempDiag/PCBOverTempDiag/EnableJudgement ==
  SysSelfCheckDownFlg : Inport
  DiagEn : Inport  Port=2
  Constant : Constant  Value=true
  Logical Operator : Logic  AllPortsSameDT=off  OutDataTypeStr=boolean
  Logical Operator1 : Logic  AllPortsSameDT=off  OutDataTypeStr=boolean
  Logical Operator2 : Logic  AllPortsSameDT=off  OutDataTypeStr=boolean
  DiagEnOut : Outport
  wires:
  Logical Operator2/1 -> DiagEnOut/1  "M_Flt_PCBOverTempDiagEn_b"
  Logical Operator/1 -> Logical Operator2/1
  SysSelfCheckDownFlg/1 -> Logical Operator/2
  DiagEn/1 -> Logical Operator1/2
  Constant/1 -> Logical Operator/1, Logical Operator1/1
  Logical Operator1/1 -> Logical Operator2/2

== system FaultCheck/FaultDiagnose/PCBTempDiag/PCBOverTempDiag/FaultLevelDeter ==
  PCBOverTempFlgOut : Inport
  FaultLevel : Inport  Port=2
  If : If  IfExpression=u1 == 0
  LowerOne : Subsystem  TreatAsAtomicUnit=on
  Merge : Merge
  Normal : Subsystem  TreatAsAtomicUnit=on
  PCBOverTempFltLevelOut : Outport
  wires:
  PCBOverTempFlgOut/1 -> If/1
  If/1 -> Normal/Action
  If/2 -> LowerOne/Action
  Normal/1(PCBOverTempFltLevel) -> Merge/1
  LowerOne/1(PCBOverTempFltLevel) -> Merge/2
  Merge/1 -> PCBOverTempFltLevelOut/1  "M_Flt_PCBOverTempFltLevelOut_u8"
  FaultLevel/1 -> LowerOne/1(FaultLevel)

== system FaultCheck/FaultDiagnose/PCBTempDiag/PCBOverTempDiag/Parameters ==
  PCBTemp : Inport
  1-D Lookup Table1 : Lookup_n-D  NumberOfTableDimensions=1  BreakpointsForDimension1=[-5:5]  BreakpointsForDimension1DataTypeStr=Inherit: Inherit from 'Breakpoint data'  IndexSearchMethod=Linear search  Table=tanh([-5:5])  TableDataTypeStr=Inherit: Inherit from 'Table data'  ExtrapMethod=Clip  UseLastTableValue=on  InternalRulePriority=Speed  OutDataTypeStr=single  RndMeth=Simplest
  Bus Creator : BusCreator  Inputs=8
  Constant : Constant  Value=C_Flt_PCBOverTempTrigTh_s32
  Constant1 : Constant  Value=C_Flt_PCBOverTempRecTh_s32
  Constant10 : Constant  Value=C_Flt_PCBOverTempRecoveryTh_u16
  Constant11 : Constant  Value=C_Flt_LevelTwo_u8
  Constant7 : Constant  Value=C_Flt_PCBOverTempDiagEn_b
  Constant8 : Constant  Value=C_Flt_PCBOverTempErrCode_u16
  Constant9 : Constant  Value=C_Flt_PCBOverTempConfirmTh_u16
  Param : Outport
  wires:
  Bus Creator/1 -> Param/1
  PCBTemp/1 -> 1-D Lookup Table1/1
  Constant/1 -> Bus Creator/1  "PCBOverTempTrigTh"
  Constant7/1 -> Bus Creator/3  "PCBOverTempDiagEn"
  Constant8/1 -> Bus Creator/4  "PCBOverTempErrCode"
  Constant9/1 -> Bus Creator/5  "PCBOverTempConfirmTh"
  Constant10/1 -> Bus Creator/6  "PCBOverTempRecoveryTh"
  Constant11/1 -> Bus Creator/7  "PCBOverTempFltLevel"
  1-D Lookup Table1/1 -> Bus Creator/8  "PCBOverTempPowerCoeff"
  Constant1/1 -> Bus Creator/2  "PCBOverTempRecTh"

== system FaultCheck/FaultDiagnose/PCBTempDiag/PCBOverTempDiag/PowerReductionCoeffDeter ==
  PCBOverTempFltLevelOut : Inport
  PowerCoeff : Inport  Port=2
  If : If  IfExpression=u1 < 2  ElseIfExpressions=u1 == 2
  If Action Subsystem : Subsystem  TreatAsAtomicUnit=on
  If Action Subsystem1 : Subsystem  TreatAsAtomicUnit=on
  If Action Subsystem2 : Subsystem  TreatAsAtomicUnit=on
  Merge : Merge  Inputs=3
  PCBOverTempPowerCoeffOut : Outport
  wires:
  PCBOverTempFltLevelOut/1 -> If/1
  If/1 -> If Action Subsystem/Action
  If/2 -> If Action Subsystem1/Action
  If/3 -> If Action Subsystem2/Action
  PowerCoeff/1 -> If Action Subsystem1/1(PowerCoeff)
  If Action Subsystem/1(Coeff) -> Merge/1
  If Action Subsystem1/1(Coeff) -> Merge/2
  If Action Subsystem2/1(Coeff) -> Merge/3
  Merge/1 -> PCBOverTempPowerCoeffOut/1  "M_Flt_PCBOverTempPowerCoeffOut_s32"

== system FaultCheck/FaultDiagnose/PhaseCurrDiag/Flt_IuOverCurrDiag/Diagnose ==
  SysSelfCheckDownFlg : Inport
  IuOCParam : Inport  Port=2
  UPhaseCurr_A : Inport  Port=3
  Bus Selector : BusSelector  OutputSignals=IuOCDiagEn
  Disable : Subsystem  TreatAsAtomicUnit=on
  Enable : Subsystem  TreatAsAtomicUnit=on
  Enable Judgement : Subsystem
  If : If  IfExpression=u1 == 0
  Merge : Merge
  IuOCFltFlg : Outport
  wires:
  IuOCParam/1 -> Bus Selector/1, Enable/1(IuOCParam)
  SysSelfCheckDownFlg/1 -> Enable Judgement/1(SysSelfCheckDownFlg)
  Enable Judgement/1(IuOCDiagEnFlg) -> If/1
  If/1 -> Disable/Action
  If/2 -> Enable/Action
  UPhaseCurr_A/1 -> Enable/2(UPhaseCurr_A)
  Merge/1 -> IuOCFltFlg/1  "M_Flt_IuOCFltFlgOut_b"
  Disable/1(IuOCFltFlg) -> Merge/1
  Enable/1(IuOCFlgDeb) -> Merge/2
  Bus Selector/1 -> Enable Judgement/2(IuOCDiagDiagEn)  "<IuOCDiagEn>"

== system FaultCheck/FaultDiagnose/PhaseCurrDiag/Flt_IuOverCurrDiag/FaultLevelDeter ==
  IuOCFltFlg : Inport
  IuOCParam : Inport  Port=2
  Bus Selector : BusSelector  OutputSignals=IuOCFltLevel
  If : If  IfExpression=u1 == 0
  Merge : Merge
  Normal : Subsystem  TreatAsAtomicUnit=on
  OverCurr : Subsystem  TreatAsAtomicUnit=on
  IuOCFltLevelOut : Outport
  wires:
  IuOCFltFlg/1 -> If/1
  If/1 -> Normal/Action
  If/2 -> OverCurr/Action
  IuOCParam/1 -> Bus Selector/1
  Bus Selector/1 -> OverCurr/1(FaultLevel)  "<IuOCFltLevel>"
  Normal/1(IuOCFltLevel) -> Merge/1
  OverCurr/1(IuOCFltLevel) -> Merge/2
  Merge/1 -> IuOCFltLevelOut/1  "M_Flt_IuOCFltLevelOut_u8"

== system FaultCheck/FaultDiagnose/PhaseCurrDiag/Flt_IuOverCurrDiag/Parameters ==
  Bus Creator : BusCreator  Inputs=8
  Constant1 : Constant  Value=C_Flt_IuOCNegLimit_s32
  Constant11 : Constant  Value=C_Flt_IuOCErrCode_u16
  Constant13 : Constant  Value=C_Flt_LevelFour_u8
  Constant2 : Constant  Value=C_Flt_PowerCoeffZero_s32
  Constant3 : Constant  Value=C_Flt_IuOCRecoveryTh_u16
  Constant6 : Constant  Value=C_Flt_IuOCDiagEn_b
  Constant7 : Constant  Value=C_Flt_IuOCPosLimit_s32
  Constant8 : Constant  Value=C_Flt_IuOCConfirmTh_u16
  IuOCParam : Outport
  wires:
  Bus Creator/1 -> IuOCParam/1
  Constant11/1 -> Bus Creator/6  "IuOCErrCode"
  Constant8/1 -> Bus Creator/3  "IuOCConfirmTh"
  Constant1/1 -> Bus Creator/2  "IuOCNegLimit"
  Constant2/1 -> Bus Creator/8  "IuOCPowerCoeff"
  Constant13/1 -> Bus Creator/7  "IuOCFltLevel"
  Constant7/1 -> Bus Creator/1  "IuOCPosLimit"
  Constant6/1 -> Bus Creator/5  "IuOCDiagEn"
  Constant3/1 -> Bus Creator/4  "IuOCRecoveryTh"

== system FaultCheck/FaultDiagnose/PhaseCurrDiag/Flt_IuOverCurrDiag/PowerReductionCoeffDeter ==
  IuOCFltLevelOut : Inport
  PowerCoeff : Inport  Port=2
  If : If  IfExpression=u1 < 2  ElseIfExpressions=u1 == 2
  If Action Subsystem : Subsystem  TreatAsAtomicUnit=on
  If Action Subsystem1 : Subsystem  TreatAsAtomicUnit=on
  If Action Subsystem2 : Subsystem  TreatAsAtomicUnit=on
  Merge : Merge  Inputs=3
  IuOCPowerCoeff : Outport
  wires:
  IuOCFltLevelOut/1 -> If/1
  If/1 -> If Action Subsystem/Action
  If/2 -> If Action Subsystem1/Action
  If/3 -> If Action Subsystem2/Action
  PowerCoeff/1 -> If Action Subsystem1/1(PowerCoeff)
  If Action Subsystem/1(Coeff) -> Merge/1
  If Action Subsystem1/1(Coeff) -> Merge/2
  If Action Subsystem2/1(Coeff) -> Merge/3
  Merge/1 -> IuOCPowerCoeff/1  "M_Flt_IuOCPowerCoeffOut_s32"

== system FaultCheck/FaultDiagnose/PhaseCurrDiag/Flt_IvOverCurrDiag/Diagnose ==
  SysSelfCheckDownFlg : Inport
  IvOCParam : Inport  Port=2
  VPhaseCurr_A : Inport  Port=3
  Bus Selector : BusSelector  OutputSignals=IvOCDiagEn
  Disable : Subsystem  TreatAsAtomicUnit=on
  Enable : Subsystem  TreatAsAtomicUnit=on
  Enable Judgement : Subsystem
  If : If  IfExpression=u1 == 0
  Merge : Merge
  IvOCFltFlg : Outport
  wires:
  Bus Selector/1 -> Enable Judgement/2(IvOCDiagDiagEn)  "<IvOCDiagEn>"
  Enable/1(IvOCFlgDeb) -> Merge/2
  Disable/1(IvOCFltFlg) -> Merge/1
  Merge/1 -> IvOCFltFlg/1  "M_Flt_IvOCFltFlgOut_b"
  VPhaseCurr_A/1 -> Enable/2(VPhaseCurr_A)
  If/2 -> Enable/Action
  If/1 -> Disable/Action
  Enable Judgement/1(IvOCDiagEnFlg) -> If/1
  SysSelfCheckDownFlg/1 -> Enable Judgement/1(SysSelfCheckDownFlg)
  IvOCParam/1 -> Enable/1(IvOCParam), Bus Selector/1

== system FaultCheck/FaultDiagnose/PhaseCurrDiag/Flt_IvOverCurrDiag/FaultLevelDeter ==
  IvOCFltFlg : Inport
  IvOCParam : Inport  Port=2
  Bus Selector : BusSelector  OutputSignals=IvOCFltLevel
  If : If  IfExpression=u1 == 0
  Merge : Merge
  Normal : Subsystem  TreatAsAtomicUnit=on
  OverCurr : Subsystem  TreatAsAtomicUnit=on
  IvOCFltLevelOut : Outport
  wires:
  Merge/1 -> IvOCFltLevelOut/1  "M_Flt_IvOCFltLevelOut_u8"
  OverCurr/1(IvOCFltLevel) -> Merge/2
  Normal/1(IvOCFltLevel) -> Merge/1
  Bus Selector/1 -> OverCurr/1(FaultLevel)  "<IvOCFltLevel>"
  IvOCParam/1 -> Bus Selector/1
  If/2 -> OverCurr/Action
  If/1 -> Normal/Action
  IvOCFltFlg/1 -> If/1

== system FaultCheck/FaultDiagnose/PhaseCurrDiag/Flt_IvOverCurrDiag/Parameters ==
  Bus Creator : BusCreator  Inputs=8
  Constant1 : Constant  Value=C_Flt_IvOCNegLimit_s32
  Constant11 : Constant  Value=C_Flt_IvOCErrCode_u16
  Constant13 : Constant  Value=C_Flt_LevelFour_u8
  Constant2 : Constant  Value=C_Flt_PowerCoeffZero_s32
  Constant3 : Constant  Value=C_Flt_IvOCRecoveryTh_u16
  Constant6 : Constant  Value=C_Flt_IvOCDiagEn_b
  Constant7 : Constant  Value=C_Flt_IvOCPosLimit_s32
  Constant8 : Constant  Value=C_Flt_IvOCConfirmTh_u16
  IvOCParam : Outport
  wires:
  Constant6/1 -> Bus Creator/5  "IvOCDiagEn"
  Constant7/1 -> Bus Creator/1  "IvOCPosLimit"
  Constant13/1 -> Bus Creator/7  "IvOCFltLevel"
  Constant2/1 -> Bus Creator/8  "IvOCPowerCoeff"
  Constant1/1 -> Bus Creator/2  "IvOCNegLimit"
  Constant8/1 -> Bus Creator/3  "IvOCConfirmTh"
  Constant11/1 -> Bus Creator/6  "IvOCErrCode"
  Bus Creator/1 -> IvOCParam/1
  Constant3/1 -> Bus Creator/4  "IvOCRecoveryTh"

== system FaultCheck/FaultDiagnose/PhaseCurrDiag/Flt_IvOverCurrDiag/PowerReductionCoeffDeter ==
  IvOCFltLevelOut : Inport
  PowerCoeff : Inport  Port=2
  If : If  IfExpression=u1 < 2  ElseIfExpressions=u1 == 2
  If Action Subsystem : Subsystem  TreatAsAtomicUnit=on
  If Action Subsystem1 : Subsystem  TreatAsAtomicUnit=on
  If Action Subsystem2 : Subsystem  TreatAsAtomicUnit=on
  Merge : Merge  Inputs=3
  IvOCPowerCoeff : Outport
  wires:
  Merge/1 -> IvOCPowerCoeff/1  "M_Flt_IvOCPowerCoeffOut_s32"
  If Action Subsystem2/1(Coeff) -> Merge/3
  If Action Subsystem1/1(Coeff) -> Merge/2
  If Action Subsystem/1(Coeff) -> Merge/1
  PowerCoeff/1 -> If Action Subsystem1/1(PowerCoeff)
  If/3 -> If Action Subsystem2/Action
  If/2 -> If Action Subsystem1/Action
  If/1 -> If Action Subsystem/Action
  IvOCFltLevelOut/1 -> If/1

== system FaultCheck/FaultDiagnose/PhaseCurrDiag/Flt_IwOverCurrDiag/Diagnose ==
  SysSelfCheckDownFlg : Inport
  IwOCParam : Inport  Port=2
  VPhaseCurr_A : Inport  Port=3
  Bus Selector : BusSelector  OutputSignals=IwOCDiagEn
  Disable : Subsystem  TreatAsAtomicUnit=on
  Enable : Subsystem  TreatAsAtomicUnit=on
  Enable Judgement : Subsystem
  If : If  IfExpression=u1 == 0
  Merge : Merge
  IwOCFltFlg : Outport
  wires:
  IwOCParam/1 -> Bus Selector/1, Enable/1(IwOCParam)
  SysSelfCheckDownFlg/1 -> Enable Judgement/1(SysSelfCheckDownFlg)
  Enable Judgement/1(IwOCDiagEnFlg) -> If/1
  If/1 -> Disable/Action
  If/2 -> Enable/Action
  VPhaseCurr_A/1 -> Enable/2(VPhaseCurr_A)
  Merge/1 -> IwOCFltFlg/1  "M_Flt_IwOCFltFlgOut_b"
  Disable/1(IwOCFltFlg) -> Merge/1
  Enable/1(IwOCFlgDeb) -> Merge/2
  Bus Selector/1 -> Enable Judgement/2(IwOCDiagDiagEn)  "<IwOCDiagEn>"

== system FaultCheck/FaultDiagnose/PhaseCurrDiag/Flt_IwOverCurrDiag/FaultLevelDeter ==
  IwOCFltFlg : Inport
  IwOCParam : Inport  Port=2
  Bus Selector : BusSelector  OutputSignals=IwOCFltLevel
  If : If  IfExpression=u1 == 0
  Merge : Merge
  Normal : Subsystem  TreatAsAtomicUnit=on
  OverCurr : Subsystem  TreatAsAtomicUnit=on
  IwOCFltLevelOut : Outport
  wires:
  IwOCFltFlg/1 -> If/1
  If/1 -> Normal/Action
  If/2 -> OverCurr/Action
  IwOCParam/1 -> Bus Selector/1
  Bus Selector/1 -> OverCurr/1(FaultLevel)  "<IwOCFltLevel>"
  Normal/1(IwOCFltLevel) -> Merge/1
  OverCurr/1(IwOCFltLevel) -> Merge/2
  Merge/1 -> IwOCFltLevelOut/1  "M_Flt_IwOCFltLevelOut_u8"

== system FaultCheck/FaultDiagnose/PhaseCurrDiag/Flt_IwOverCurrDiag/Parameters ==
  Bus Creator : BusCreator  Inputs=8
  Constant1 : Constant  Value=C_Flt_IwOCNegLimit_s32
  Constant11 : Constant  Value=C_Flt_IwOCErrCode_u16
  Constant13 : Constant  Value=C_Flt_LevelFour_u8
  Constant2 : Constant  Value=C_Flt_PowerCoeffZero_s32
  Constant3 : Constant  Value=C_Flt_IwOCRecoveryTh_u16
  Constant6 : Constant  Value=C_Flt_IwOCDiagEn_b
  Constant7 : Constant  Value=C_Flt_IwOCPosLimit_s32
  Constant8 : Constant  Value=C_Flt_IwOCConfirmTh_u16
  IwOCParam : Outport
  wires:
  Bus Creator/1 -> IwOCParam/1
  Constant11/1 -> Bus Creator/6  "IwOCErrCode"
  Constant8/1 -> Bus Creator/3  "IwOCConfirmTh"
  Constant1/1 -> Bus Creator/2  "IwOCNegLimit"
  Constant2/1 -> Bus Creator/8  "IwOCPowerCoeff"
  Constant13/1 -> Bus Creator/7  "IwOCFltLevel"
  Constant7/1 -> Bus Creator/1  "IwOCPosLimit"
  Constant6/1 -> Bus Creator/5  "IwOCDiagEn"
  Constant3/1 -> Bus Creator/4  "IwOCRecoveryTh"

== system FaultCheck/FaultDiagnose/PhaseCurrDiag/Flt_IwOverCurrDiag/PowerReductionCoeffDeter ==
  IwOCFltLevelOut : Inport
  PowerCoeff : Inport  Port=2
  If : If  IfExpression=u1 < 2  ElseIfExpressions=u1 == 2
  If Action Subsystem : Subsystem  TreatAsAtomicUnit=on
  If Action Subsystem1 : Subsystem  TreatAsAtomicUnit=on
  If Action Subsystem2 : Subsystem  TreatAsAtomicUnit=on
  Merge : Merge  Inputs=3
  IwOCPowerCoeff : Outport
  wires:
  IwOCFltLevelOut/1 -> If/1
  If/1 -> If Action Subsystem/Action
  If/2 -> If Action Subsystem1/Action
  If/3 -> If Action Subsystem2/Action
  PowerCoeff/1 -> If Action Subsystem1/1(PowerCoeff)
  If Action Subsystem/1(Coeff) -> Merge/1
  If Action Subsystem1/1(Coeff) -> Merge/2
  If Action Subsystem2/1(Coeff) -> Merge/3
  Merge/1 -> IwOCPowerCoeff/1  "M_Flt_IwOCPowerCoeffOut_s32"

== system FaultCheck/FaultDiagnose/UdcLowerOneDiag/Diagnose/Disable ==
  Action Port : ActionPort  ActionPortLabel=if(u1 == 0)
  Constant : Constant  Value=C_Flt_NoErr_b
  UdcLowerOneFltDeb : Outport
  wires:
  Constant/1 -> UdcLowerOneFltDeb/1

== system FaultCheck/FaultDiagnose/UdcLowerOneDiag/Diagnose/NormalDiag ==
  Udc : Inport
  Parameter : Inport  Port=2
  Action Port : ActionPort  ActionPortLabel=else
  Bus Selector : BusSelector  OutputSignals=UdcLowerOneConfirmTh,UdcLowerOneRecoveryTh,UdcLowerOneTrigTh,UdcLowerOneRecTh
  DebounceRecInTwo : YS_UserDefined_Library/Fault/DebounceRecInTwo  SystemSampleTime=-1  VariantActivationTime=update diagram  Latency=0  AutoFrameSizeCalculation=off
      settings: SourceProductName=YS
  Relational Operator : RelationalOperator  Operator=>  OutDataTypeStr=boolean  RndMeth=Simplest  InputSameDT=off
  Relational Operator1 : RelationalOperator  Operator=>  OutDataTypeStr=boolean  RndMeth=Simplest  InputSameDT=off
  Signal Copy : SignalConversion  OverrideOpt=off
  UdcLowerOneFltDeb : Outport
  wires:
  Parameter/1 -> Bus Selector/1
  Bus Selector/1 -> DebounceRecInTwo/1  "<UdcLowerOneConfirmTh>"
  Bus Selector/2 -> DebounceRecInTwo/2  "<UdcLowerOneRecoveryTh>"
  DebounceRecInTwo/1 -> Signal Copy/1  "M_Flt_UdcLowerOneFltFlgDeb_b"
  Relational Operator/1 -> DebounceRecInTwo/3  "M_Flt_UdcLowerOneFltFlgUnDeb_b"
  Signal Copy/1 -> UdcLowerOneFltDeb/1
  Bus Selector/3 -> Relational Operator/1  "<UdcLowerOneTrigTh>"
  Udc/1 -> Relational Operator1/1, Relational Operator/2
  Bus Selector/4 -> Relational Operator1/2  "<UdcLowerOneRecTh>"
  Relational Operator1/1 -> DebounceRecInTwo/4  "M_Flt_UdcLowerOneRecFlgUnDeb_b"

== system FaultCheck/FaultDiagnose/UdcLowerOneDiag/FaultLevelDeter/LowerOne ==
  FaultLevel : Inport
  Action Port : ActionPort  ActionPortLabel=else
  UdcLowerOneFltLevel : Outport
  wires:
  FaultLevel/1 -> UdcLowerOneFltLevel/1

== system FaultCheck/FaultDiagnose/UdcLowerOneDiag/FaultLevelDeter/Normal ==
  Action Port : ActionPort  ActionPortLabel=if(u1 == 0)
  Constant : Constant  Value=C_Flt_LevelZero_u8
  UdcLowerOneFltLevel : Outport
  wires:
  Constant/1 -> UdcLowerOneFltLevel/1

== system FaultCheck/FaultDiagnose/UdcLowerOneDiag/PowerReductionCoeffDeter/If Action Subsystem ==
  Action Port : ActionPort  ActionPortLabel=if(u1 < 2)
  Constant : Constant  Value=C_Flt_PowerCoeffOne_s32
  Coeff : Outport
  wires:
  Constant/1 -> Coeff/1

== system FaultCheck/FaultDiagnose/UdcLowerOneDiag/PowerReductionCoeffDeter/If Action Subsystem1 ==
  PowerCoeff : Inport
  Action Port : ActionPort  ActionPortLabel=elseif(u1 == 2)
  Coeff : Outport
  wires:
  PowerCoeff/1 -> Coeff/1

== system FaultCheck/FaultDiagnose/UdcLowerOneDiag/PowerReductionCoeffDeter/If Action Subsystem2 ==
  Action Port : ActionPort  ActionPortLabel=else
  Constant : Constant  Value=C_Flt_PowerCoeffZero_s32
  Coeff : Outport
  wires:
  Constant/1 -> Coeff/1
